simulink model "Greenhouse_1stPoint"  (R2024a)
settings: Solver=VariableStepAuto  StartTime=0.0  StopTime=H  RelTol=1e-3
values from neighbouring files (symbols this model uses):
  C_f1 = c_f * m_f1    (= 1846687500)    [init.m]
  C_f2 = c_f * m_f2    (= 492450000)    [init.m]
  kaf1 = t_t * Sm1_ext    (= 4731)    [init.m]
  kaf2 = t_t * Sm2_ext    (= 1311)    [init.m]
  kaf_int = t_t * Sm_int    (= 171)    [init.m]
  theta0_a = 100    [init.m]
  Ts = 1    [init.m]
  var_wf1 = 1    [init.m]
  var_wf2 = 1    [init.m]
settings Model: Creator=mrnel  LastModifiedBy=dadug
settings ModelReferenceCC: EnableRefExpFcnMdlSchedulingChecks=on
settings RTWCC: GPUComputeCapability=3.5

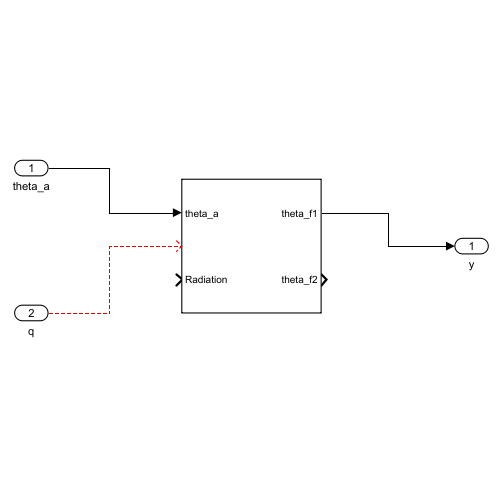
[thumbnail: Simulink's stored preview of the top-level diagram]
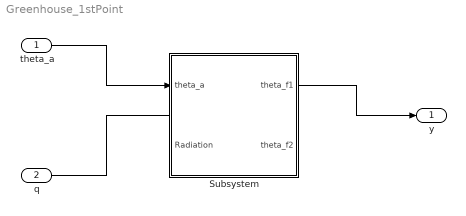
== system Greenhouse_1stPoint ==
  theta_a : Inport
  q : Inport  Port=2
  Subsystem : Subsystem
  y : Outport
  wires:
  theta_a/1 -> Subsystem/1(theta_a)
  q/1 -> ?
  Subsystem/1(theta_f1) -> y/1

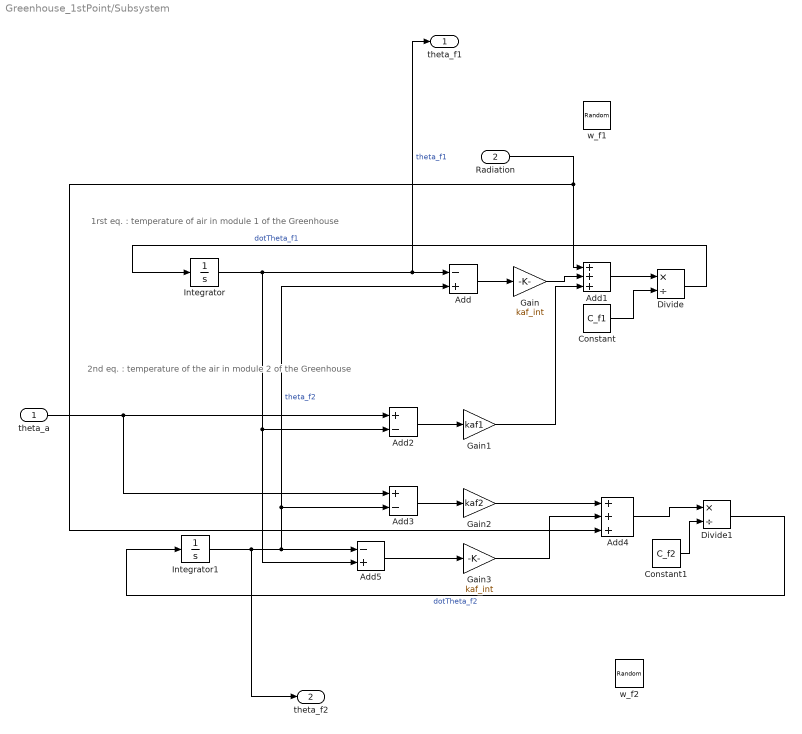
== system Greenhouse_1stPoint/Subsystem ==
  note: 2nd eq. : temperature of the air in module 2 of the Greenhouse
  note: 1rst eq. : temperature of air in module 1 of the Greenhouse
  theta_a : Inport
  Radiation : Inport  Port=2
  Add : Sum  Inputs=-+
  Add1 : Sum  Inputs=+++
  Add2 : Sum  Inputs=+-
  Add3 : Sum  Inputs=+-
  Add4 : Sum  Inputs=+++
  Add5 : Sum  Inputs=-+
  Constant : Constant  Value=C_f1
  Constant1 : Constant  Value=C_f2
  Divide : Product  Inputs=*/
  Divide1 : Product  Inputs=*/
  Gain : Gain  Gain=kaf_int
  Gain1 : Gain  Gain=kaf1
  Gain2 : Gain  Gain=kaf2
  Gain3 : Gain  Gain=kaf_int
  Integrator : Integrator  InitialCondition=theta0_a
  Integrator1 : Integrator  InitialCondition=theta0_a
  w_f1 : RandomNumber  Variance=var_wf1  SampleTime=Ts
  w_f2 : RandomNumber  Variance=var_wf2  SampleTime=Ts
  theta_f1 : Outport
  theta_f2 : Outport  Port=2
  wires:
  Divide/1 -> Integrator/1  "dotTheta_f1"
  Add2/1 -> Gain1/1
  Add1/1 -> Divide/1
  Integrator/1 -> Add5/2, Add2/2, theta_f1/1, Add/1  "theta_f1"
  Add/1 -> Gain/1
  Constant1/1 -> Divide1/2
  Constant/1 -> Divide/2
  Add3/1 -> Gain2/1
  Add4/1 -> Divide1/1
  Radiation/1 -> Add4/3, Add1/1
  theta_a/1 -> Add3/1, Add2/1
  Gain/1 -> Add1/2
  Gain1/1 -> Add1/3
  Gain2/1 -> Add4/1
  Integrator1/1 -> theta_f2/1, Add3/2, Add/2, Add5/1  "theta_f2"
  Add5/1 -> Gain3/1
  Gain3/1 -> Add4/2
  Divide1/1 -> Integrator1/1  "dotTheta_f2"
